simulink model "monopod_model"  (R2022a)
settings: Solver=FixedStepAuto  StartTime=0.0  StopTime=10  FixedStep=1e-4  RelTol=1e-3
StopFcn:
  | t_sim = out.tout
  | x_sim = out.logsout{1}.Values.Data
  | 
  | monoplot(t_sim,x_sim)
values from neighbouring files (symbols this model uses):
  g = 9.81    [monopod_controller_parameter.sldd]
  I_1 = 0.1    [monopod_controller_parameter.sldd]
  I_2 = 0.1    [monopod_controller_parameter.sldd]
  I_body = 0.1    [monopod_controller_parameter.sldd]
  l_1 = 0.16    [monopod_controller_parameter.sldd]
  l_2 = 0.16    [monopod_controller_parameter.sldd]
  m_1 = 0.158    [monopod_controller_parameter.sldd]
  m_2 = 0.062    [monopod_controller_parameter.sldd]
  m_body = 0.1    [monopod_controller_parameter.sldd]
settings Model: DataDictionary=monopod_model_parameter.sldd  EnableAccessToBaseWorkspace=off  PacingRate=0.001000  Creator=chris  LastModifiedBy=chris
settings DebuggingCC: UnconnectedInputMsg=warning  UnconnectedOutputMsg=warning  UnconnectedLineMsg=warning
settings RTWCC: DLArmComputeVersion=19.05

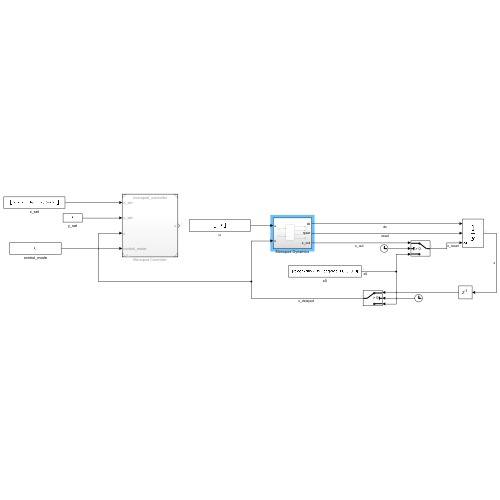
[thumbnail: Simulink's stored preview of the top-level diagram]
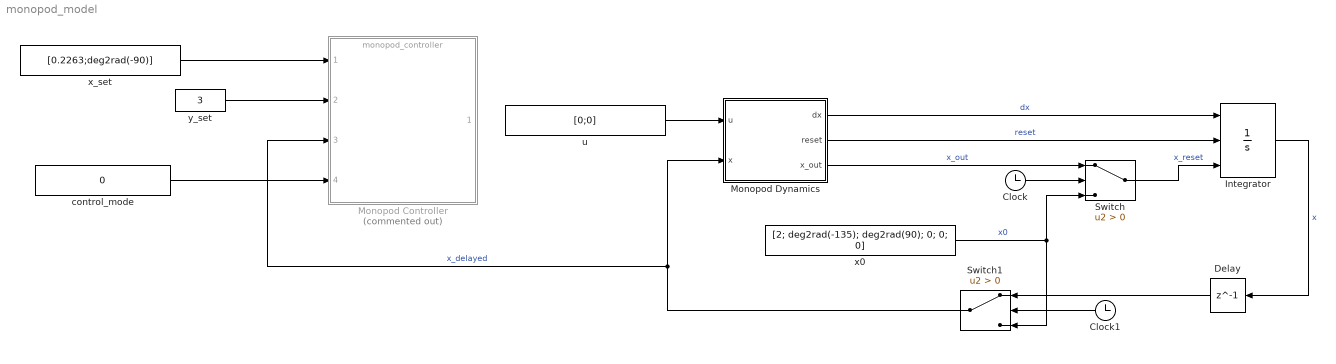
== system monopod_model ==
  Clock : Clock
  Clock1 : Clock
  Delay : Delay  DelayLength=1
  Integrator : Integrator  ExternalReset=level  InitialConditionSource=external
  Monopod Controller : ModelReference  Commented=on  ModelNameDialog=monopod_controller.slx  SimulationMode=Normal  ModelReferenceVersion=1.133
  Monopod Dynamics : Subsystem
  Switch : Switch  Criteria=u2 > Threshold  SaturateOnIntegerOverflow=off  InputSameDT=off
  Switch1 : Switch  Criteria=u2 > Threshold  SaturateOnIntegerOverflow=off  InputSameDT=off
  control_mode : Constant  Value=0
  u : Constant  Value=[0;0]
  x0 : Constant  Value=[2; deg2rad(-135); deg2rad(90); 0; 0; 0]
  x_set : Constant  Value=[0.2263;deg2rad(-90)]
  y_set : Constant  Value=3
  wires:
  Monopod Dynamics/2(reset) -> Integrator/2  "reset"
  x0/1 -> Switch/3, Switch1/3  "x0"
  Clock/1 -> Switch/2
  Switch/1 -> Integrator/3  "x_reset"
  Monopod Dynamics/3(x_out) -> Switch/1  "x_out"
  Clock1/1 -> Switch1/2
  Integrator/1 -> Delay/1  "x"
  Switch1/1 -> Monopod Controller/3, Monopod Dynamics/2(x)  "x_delayed"
  Delay/1 -> Switch1/1
  x_set/1 -> Monopod Controller/1
  Monopod Dynamics/1(dx) -> Integrator/1  "dx"
  control_mode/1 -> Monopod Controller/4
  y_set/1 -> Monopod Controller/2
  u/1 -> Monopod Dynamics/1(u)

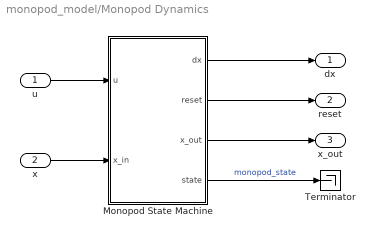
== system monopod_model/Monopod Dynamics ==
  u : Inport
  x : Inport  Port=2  PortDimensions=6
  Monopod State Machine : Stateflow chart  TreatAsAtomicUnit=on
  Terminator : Terminator
  dx : Outport  PortDimensions=6
  reset : Outport  Port=2
  x_out : Outport  Port=3
  wires:
  x/1 -> Monopod State Machine/2(x_in)
  u/1 -> Monopod State Machine/1(u)
  Monopod State Machine/1(dx) -> dx/1
  Monopod State Machine/2(reset) -> reset/1
  Monopod State Machine/3(x_out) -> x_out/1
  Monopod State Machine/4(state) -> Terminator/1  "monopod_state"

== stateflow chart monopod_model/Monopod Dynamics/Monopod State Machine ==
  state Flight_Phase
    entry:
    reset = false;
    state = "flight"
    x = x_in;
    y_foot = get_c(0,x);
    during:
    x = x_in;
    dx = get_dyn_flight(0,x,u);
    y_foot = get_c(0,x);
  state Stance_Phase
    entry:
    state = "stance"
    dx = get_dyn_stance(0,x,u);
    lambda = get_lambda(x,u);
    during:
    x = x_in;
    dx = get_dyn_stance(0,x,u);
    lambda = get_lambda(x,u)
  state Impact_Phase
    entry:
    state = "impact"
    x(4:6) = get_impact(x);
    x_out = x;
  Stance_Phase -> Flight_Phase : [ abs(lambda(2)) <= 0.001 ]{ reset = true; }
  (default) -> Flight_Phase
  Flight_Phase -> Impact_Phase : [ y_foot <= 0]{ reset = true; }
  Impact_Phase -> Stance_Phase : { reset = false; }
  data: u input; x_in input; dx output; y_foot local; x local; reset output =false; x_out output; state output; lambda local; I_1 parameter; I_2 parameter; I_body parameter; l_1 parameter; l_2 parameter; m_1 parameter; m_2 parameter; m_body parameter; g parameter
